simulink model "mtpa"  (R2022b)
settings: Solver=VariableStepAuto  StartTime=0.0  StopTime=1  RelTol=1e-3
undefined symbols (not defined in the file): ibez, Ld, Ld_norm, Lq, Lq_norm, magnitude, phi_m, phi_m_norm
settings Model: Creator=ltnbda  LastModifiedBy=ltnbda

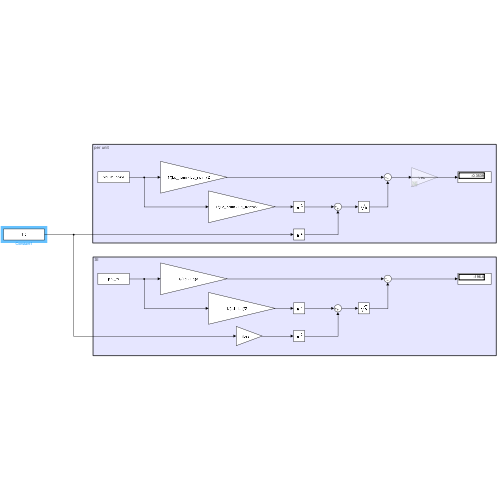
[thumbnail: Simulink's stored preview of the top-level diagram]
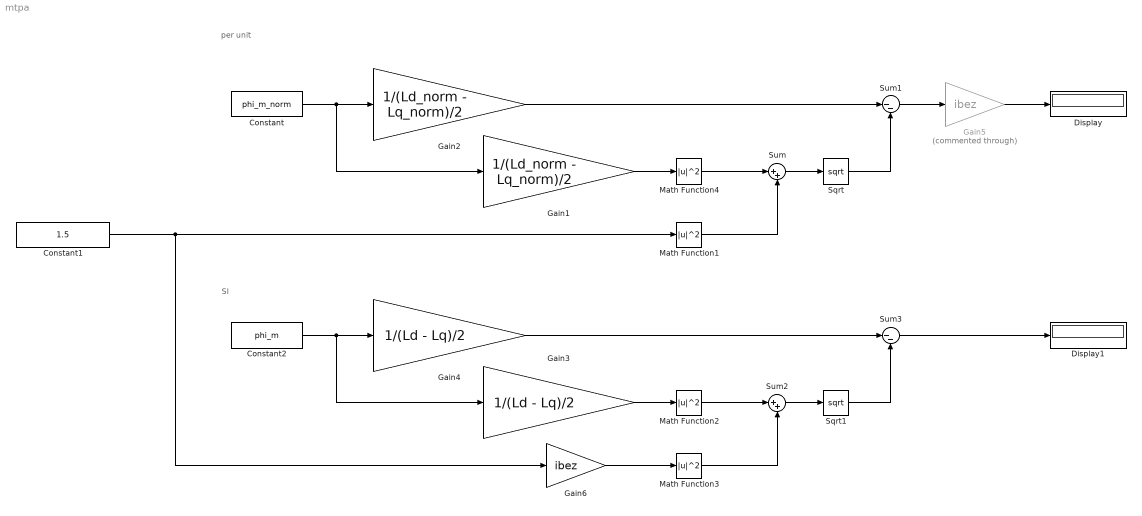
== system mtpa ==
  note: SI
  note: per unit
  Constant : Constant  Value=phi_m_norm
  Constant1 : Constant  Value=1.5
  Constant2 : Constant  Value=phi_m
  Display : Display
  Display1 : Display
  Gain1 : Gain  Gain=1/(Ld_norm - Lq_norm)/2
  Gain2 : Gain  Gain=1/(Ld_norm - Lq_norm)/2
  Gain3 : Gain  Gain=1/(Ld - Lq)/2
  Gain4 : Gain  Gain=1/(Ld - Lq)/2
  Gain5 : Gain  Commented=through  Gain=ibez
  Gain6 : Gain  Gain=ibez
  Math Function{1..4} (4 alike) : Math  Operator=magnitude^2  SignedPower=on
  Sqrt : Sqrt
  Sqrt1 : Sqrt
  Sum : Sum  Inputs=|++
  Sum1 : Sum  Inputs=|--
  Sum2 : Sum  Inputs=|++
  Sum3 : Sum  Inputs=|--
  wires:
  Constant1/1 -> Gain6/1, Math Function1/1
  Sum/1 -> Sqrt/1
  Sqrt/1 -> Sum1/2
  Constant/1 -> Gain1/1, Gain2/1
  Sum1/1 -> Gain5/1
  Gain2/1 -> Sum1/1
  Gain1/1 -> Math Function4/1
  Math Function1/1 -> Sum/2
  Math Function3/1 -> Sum2/2
  Gain3/1 -> Math Function2/1
  Gain4/1 -> Sum3/1
  Sum3/1 -> Display1/1
  Constant2/1 -> Gain3/1, Gain4/1
  Sqrt1/1 -> Sum3/2
  Sum2/1 -> Sqrt1/1
  Gain6/1 -> Math Function3/1
  Gain5/1 -> Display/1
  Math Function2/1 -> Sum2/1
  Math Function4/1 -> Sum/1
